simulink model "untitled"  (R2022a)
settings: Solver=VariableStepAuto  StartTime=0.0  StopTime=10.0  RelTol=1e-3
settings Model: Creator=Orkun  LastModifiedBy=Orkun

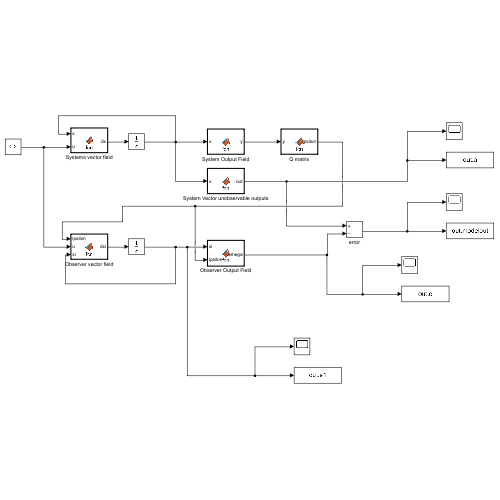
[thumbnail: Simulink's stored preview of the top-level diagram]
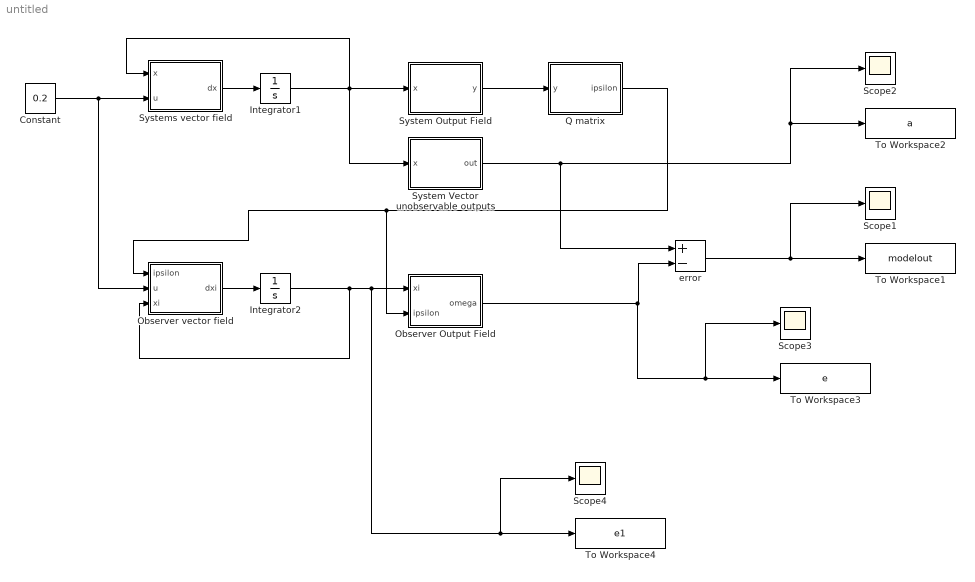
== system untitled ==
  Constant : Constant  Value=0.2
  Integrator1 : Integrator  InitialCondition=[0;0;0;0.5]
  Integrator2 : Integrator  InitialCondition=[0;0]
  Observer Output Field : MATLAB Function  TreatAsAtomicUnit=on
  Observer vector field : MATLAB Function  TreatAsAtomicUnit=on
  Q matrix : MATLAB Function  TreatAsAtomicUnit=on
  Scope{1..4} (4 alike) : Scope
  System Output Field : MATLAB Function  TreatAsAtomicUnit=on
  System Vector unobservable outputs : MATLAB Function  TreatAsAtomicUnit=on
  Systems vector field : MATLAB Function  TreatAsAtomicUnit=on
  To Workspace1 : ToWorkspace  VariableName=modelout  SaveFormat=Timeseries  SampleTime=-1
  To Workspace2 : ToWorkspace  VariableName=a  SaveFormat=Timeseries  SampleTime=-1
  To Workspace3 : ToWorkspace  VariableName=e  SaveFormat=Timeseries  SampleTime=-1
  To Workspace4 : ToWorkspace  VariableName=e1  SaveFormat=Timeseries  SampleTime=-1
  error : Sum  Inputs=+-
  wires:
  Integrator2/1 -> Observer vector field/3(xi), Scope4/1, To Workspace4/1, Observer Output Field/1(xi)
  Constant/1 -> Systems vector field/2(u), Observer vector field/2(u)
  Observer Output Field/1(omega) -> Scope3/1, To Workspace3/1, error/2
  Observer vector field/1(dxi) -> Integrator2/1
  System Vector unobservable outputs/1(out) -> Scope2/1, To Workspace2/1, error/1
  error/1 -> Scope1/1, To Workspace1/1
  Integrator1/1 -> System Vector unobservable outputs/1(x), Systems vector field/1(x), System Output Field/1(x)
  Q matrix/1(ipsilon) -> Observer Output Field/2(ipsilon), Observer vector field/1(ipsilon)
  Systems vector field/1(dx) -> Integrator1/1
  System Output Field/1(y) -> Q matrix/1(y)

== matlab function untitled/System Output Field ==
  data: x input; y output
function y = fcn(x)

C = [1, 0, 0, 0; 0, 1, 0, 0];
y = C*x;

== matlab function untitled/Q matrix ==
  data: y input; ipsilon output
function ipsilon = fcn(y)

ipsilon = [1, 0; 0, 1]*y;

== matlab function untitled/Observer Output Field ==
  data: xi input; omega output; ipsilon input
function omega = fcn(xi, ipsilon)

L = [0, -0.0475; 0, 2.7];

omega = xi + L*ipsilon;

== matlab function untitled/Observer vector field ==
  data: ipsilon input; u input; dxi output; xi input
function dxi = fcn(ipsilon,u, xi)
F = [-16.300, 0.0475; -967.95, -2.7];
G = [33.3333; 0];
H = [-0.5622, 0.8753; 31.9507, 40.2604];
dxi = F*xi + H*ipsilon + G*u;

== matlab function untitled/System Vector unobservable outputs ==
  data: x input; out output
function out = fcn(x)

out = [0, 0, 1, 0; 0, 0, 0, 1]*x;

== matlab function untitled/Systems vector field ==
  data: x input; u input; dx output
function dx = fcn(x,u)

A = [0, 1, 0, 0; -11.8336, -0.5779, 358.5000, 1; 0, 0, -33.3333, 0; 0, 0, 0, 0];
B = [0; 0; 33.3333; 0];


dx = (A*x) + (B*u);
